simulink model "systune_darko"  (R2021b)
settings: Solver=VariableStepAuto  StartTime=0.0  StopTime=50  RelTol=1e-3
values from neighbouring files (symbols this model uses):
  C_control = [C(1:7,:);C(9:12,:)]    [main.m]
  drone = generateDarko()    [main.m]
  H_complet = solution(5:6,:)    [main.m]
  H_val = H_val.D    [main.m]
  initial_state = [p_initial; v_initial; q_initial; omega_initial]    [main.m]
  K_val = K_val.D    [main.m]
  Ki_complet = solution(1:4,:)    [main.m]
  u_eq_ = u_eq    [main.m]
  w = [0;0;0]    [main.m]
  x_eq_ = [[0; 0; 0]; [0; 0; 0]; [0; 0]; [0; 0; 0]]    [main.m]
libraries: simulink_extras x14, sharedtransform x2
settings Model: Creator=florian  LastModifiedBy=florian
settings SolverCC: AlgebraicLoopSolver=TrustRegion
settings DebuggingCC: SFMachineParentedDataDiag=warning

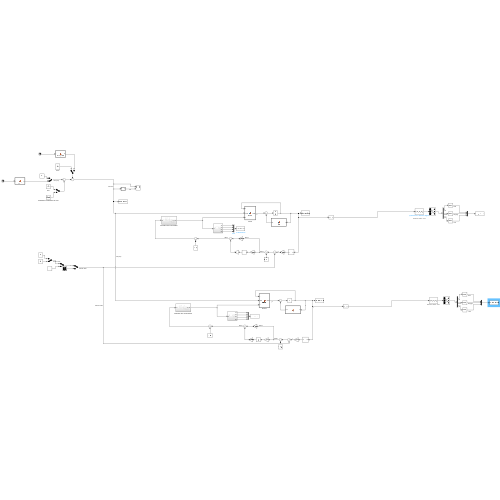
[thumbnail: Simulink's stored preview of the top-level diagram]
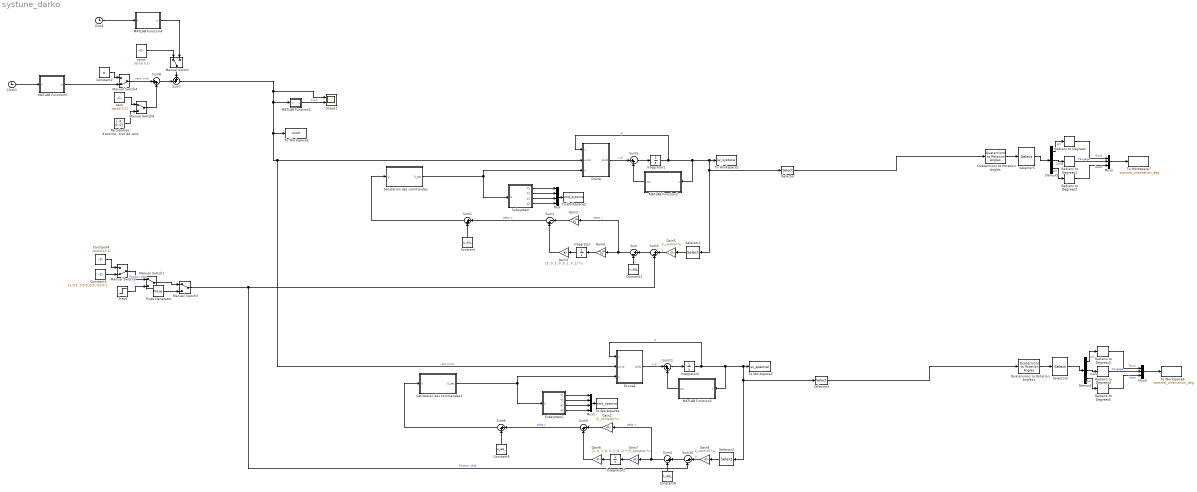
== system systune_darko ==
  Clock : Clock
  Clock1 : Clock
  Constant : Constant  Value=u_eq_
  Constant1 : Constant  Value=x_eq_
  Constant2 : Constant  Value=w
  Constant3 : Constant  Value=[1;0;1; 0;0;0; 0;0; 0;0;0;]
  Constant4 : Constant  Value=zeros(11,1)
  Constant5 : Constant  Value=u_eq_
  Constant6 : Constant  Value=x_eq_
  Demux1 : Demux  Outputs=3
  Demux5 : Demux  Outputs=3
  Drone : MATLAB Function  TreatAsAtomicUnit=on
  Drone1 : MATLAB Function  TreatAsAtomicUnit=on
  Gain1 : Gain  Gain=K_val  Multiplication=Matrix(K*u) (u vector)
  Gain2 : Gain  Gain=Ki_complet  Multiplication=Matrix(K*u) (u vector)
  Gain3 : Gain  Gain=[1, 0; 1, 0; 0, 1; 0, 1]  Multiplication=Matrix(K*u) (u vector)
  Gain4 : Gain  Gain=H_val  Multiplication=Matrix(K*u) (u vector)
  Gain5 : Gain  Gain=C_control  Multiplication=Matrix(K*u) (u vector)
  Gain6 : Gain  Gain=[1, 0; 1, 0; 0, 1; 0, 1]  Multiplication=Matrix(K*u) (u vector)
  Gain7 : Gain  Gain=H_complet  Multiplication=Matrix(K*u) (u vector)
  Gain8 : Gain  Gain=C_control  Multiplication=Matrix(K*u) (u vector)
  Integrator : Integrator  InitialCondition=zeros(1,2)
  Integrator1 : Integrator  InitialCondition=initial_state
  Integrator2 : Integrator  InitialCondition=zeros(1,2)
  Integrator3 : Integrator  InitialCondition=initial_state
  MATLAB Function1 : MATLAB Function  TreatAsAtomicUnit=on
  MATLAB Function2 : MATLAB Function  TreatAsAtomicUnit=on
  MATLAB Function3 : MATLAB Function  TreatAsAtomicUnit=on
  MATLAB Function4 : MATLAB Function  TreatAsAtomicUnit=on
  MATLAB Function5 : MATLAB Function  TreatAsAtomicUnit=on
  Manual Switch{,1,3,6} (4 alike) : ManualSwitch
  Manual Switch4 : ManualSwitch  CurrentSetting=0
  Manual Switch5 : ManualSwitch  CurrentSetting=0
  Mux : Mux
  Mux1 : Mux
  Mux2 : Mux  Inputs=3
  Mux3 : Mux  Inputs=3
  Pertubation d'estimation de vent : Constant  Value=[-3; 0; 0]
  Pulse Generator : DiscretePulseGenerator  PulseType=Time based  Amplitude=[0;0;-5; 0;0;0; 0;0; 0;0;0]  Period=5  PulseWidth=50
  Quaternions to Rotation Angles : sharedtransform/Quaternions to Rotation Angles  rotationOrder=ZXY  aMode=aMode
      settings: SourceProductBaseCode=AE,PW,DR,MT,UV,VE
  Quaternions to Rotation Angles1 : sharedtransform/Quaternions to Rotation Angles  rotationOrder=ZXY  aMode=aMode
      settings: SourceProductBaseCode=AE,PW,DR,MT,UV,VE
  Radians to Degrees{,1..5} (6 alike) : simulink_extras/Transformations/Radians to Degrees
  Satutation des commandes : Subsystem
  Satutation des commandes1 : Subsystem
  Scope1 : Scope  NumInputPorts=2
  Selector : Selector  InputPortWidth=13  IndexOptions=Index vector (dialog)  Indices=[7:10]  OutputSizes=1
  Selector1 : Selector  InputPortWidth=13  IndexOptions=Index vector (dialog)  Indices=[1:6 8:13]  OutputSizes=1
  Selector2 : Selector  InputPortWidth=13  IndexOptions=Index vector (dialog)  Indices=[1:6 8:13]  OutputSizes=1
  Selector3 : Selector  InputPortWidth=3  IndexOptions=Index vector (dialog)  Indices=[2 3 1]  OutputSizes=1
  Selector4 : Selector  InputPortWidth=13  IndexOptions=Index vector (dialog)  Indices=[7:10]  OutputSizes=1
  Selector5 : Selector  InputPortWidth=3  IndexOptions=Index vector (dialog)  Indices=[2 3 1]  OutputSizes=1
  Step1 : Step  Time=35  Before=zeros(11,1)  After=[-0.1;0;0; 0;0;0; 0;0; 0;0;0]  SampleTime=0
  Subsystem : Subsystem
  Subsystem1 : Subsystem
  Sum{,3..4,10} (4 alike) : Sum  Inputs=|+-
  Sum{1,5..6,8,11} (5 alike) : Sum  Inputs=|++
  Sum2 : Sum  Inputs=|-+
  Sum7 : Sum  Inputs=++|
  Sum9 : Sum  Inputs=|-+
  To Workspace1 : ToWorkspace  VariableName=sv_systune  SampleTime=-1
  To Workspace2 : ToWorkspace  VariableName=cmd_systune  SampleTime=-1
  To Workspace3 : ToWorkspace  VariableName=sv_spectral  SampleTime=-1
  To Workspace4 : ToWorkspace  VariableName=cmd_spectral  SampleTime=-1
  To Workspace5 : ToWorkspace  VariableName=wind  SampleTime=-1
  To Workspace6 : ToWorkspace  VariableName=spectral_orientation_deg  SampleTime=-1
  To Workspace7 : ToWorkspace  VariableName=systune_orientation_deg  SampleTime=-1
  zero : Constant  Value=zeros(3,1)
  zeros : Constant  Value=zeros(3,1)
  wires:
  Sum5/1 -> Integrator1/1
  MATLAB Function2/1(cor) -> Sum5/2
  Drone/1(dxdt) -> Sum5/1  "x_d"
  Constant1/1 -> Sum/2
  Sum1/1 -> Satutation des commandes/1(U)
  Integrator/1 -> Gain3/1
  Sum/1 -> Gain4/1, Gain1/1  "delta x"
  Gain4/1 -> Integrator/1
  Gain1/1 -> Sum2/1
  Selector1/1 -> Gain5/1
  Gain5/1 -> Sum3/1  "y"
  Sum3/1 -> Sum/1
  Gain3/1 -> Sum2/2
  MATLAB Function5/1(w) -> Manual Switch4/2
  Constant2/1 -> Manual Switch4/1
  MATLAB Function1/1(y) -> Scope1/2  "kmh"
  Step1/1 -> Manual Switch1/2
  Pulse Generator/1 -> Manual Switch3/2
  Manual Switch1/1 -> Manual Switch3/1
  Clock/1 -> MATLAB Function4/1(t)
  Constant3/1 -> Manual Switch5/2
  Manual Switch5/1 -> Manual Switch1/1  "Position cible"
  Constant4/1 -> Manual Switch5/1
  Integrator1/1 -> Drone/1(x), To Workspace1/1, Selector1/1, Selector/1, MATLAB Function2/1(x)  "p"
  Subsystem/1(T1) -> Mux/1
  Subsystem/3(d1) -> Mux/3
  Satutation des commandes/1(U_sat) -> Subsystem/1(U), Drone/3(u)
  Subsystem/2(T2) -> Mux/2
  Subsystem/4(d2) -> Mux/4
  Manual Switch/1 -> Sum7/1
  MATLAB Function4/1(w) -> Manual Switch/2
  zeros/1 -> Manual Switch/1
  Sum8/1 -> Sum7/2
  Manual Switch4/1 -> Sum8/1  "vent (m/s)"
  Pertubation d'estimation de vent/1 -> Manual Switch6/2
  Manual Switch6/1 -> Sum8/2
  zero/1 -> Manual Switch6/1
  Constant/1 -> Sum1/2
  Sum2/1 -> Sum1/1  "delta u"
  Mux/1 -> To Workspace2/1
  Subsystem1/2(T2) -> Mux1/2
  Sum4/1 -> Gain7/1, Gain2/1  "delta x"
  Drone1/1(dxdt) -> Sum11/1  "x_d"
  Sum11/1 -> Integrator3/1
  Manual Switch3/1 -> Sum3/2, Sum10/2  "Position cible"
  Selector2/1 -> Gain8/1
  Constant5/1 -> Sum6/2
  Integrator2/1 -> Gain6/1
  Satutation des commandes1/1(U_sat) -> Subsystem1/1(U), Drone1/3(u)
  Sum7/1 -> To Workspace5/1, Drone1/2(wind), Drone/2(wind), MATLAB Function1/1(u), Scope1/1  "vent (m/s)"
  Subsystem1/4(d2) -> Mux1/4
  Mux1/1 -> To Workspace4/1
  Subsystem1/3(d1) -> Mux1/3
  Subsystem1/1(T1) -> Mux1/1
  Gain6/1 -> Sum9/2
  Gain8/1 -> Sum10/1  "y"
  Constant6/1 -> Sum4/2
  MATLAB Function3/1(cor) -> Sum11/2
  Sum6/1 -> Satutation des commandes1/1(U)
  Gain2/1 -> Sum9/1
  Gain7/1 -> Integrator2/1
  Sum9/1 -> Sum6/1  "delta u"
  Sum10/1 -> Sum4/1
  Clock1/1 -> MATLAB Function5/1(t)
  Radians to Degrees/1 -> Mux2/1  "Rouli"
  Quaternions to Rotation Angles/1 -> Selector3/1
  Demux5/3 -> Radians to Degrees2/1  "psi"
  Demux5/2 -> Radians to Degrees1/1  "theta"
  Demux5/1 -> Radians to Degrees/1  "phi"
  Radians to Degrees1/1 -> Mux2/2  "Tangage"
  Selector/1 -> Quaternions to Rotation Angles/1
  Mux2/1 -> To Workspace7/1
  Radians to Degrees2/1 -> Mux2/3  "Lacet"
  Selector3/1 -> Demux5/1
  Radians to Degrees4/1 -> Mux3/2  "Tangage"
  Radians to Degrees3/1 -> Mux3/1  "Rouli"
  Selector4/1 -> Quaternions to Rotation Angles1/1
  Demux1/3 -> Radians to Degrees5/1  "psi"
  Selector5/1 -> Demux1/1
  Integrator3/1 -> Drone1/1(x), To Workspace3/1, Selector4/1, Selector2/1, MATLAB Function3/1(x)  "p"
  Radians to Degrees5/1 -> Mux3/3  "Lacet"
  Quaternions to Rotation Angles1/1 -> Selector5/1
  Mux3/1 -> To Workspace6/1
  Demux1/2 -> Radians to Degrees4/1  "theta"
  Demux1/1 -> Radians to Degrees3/1  "phi"

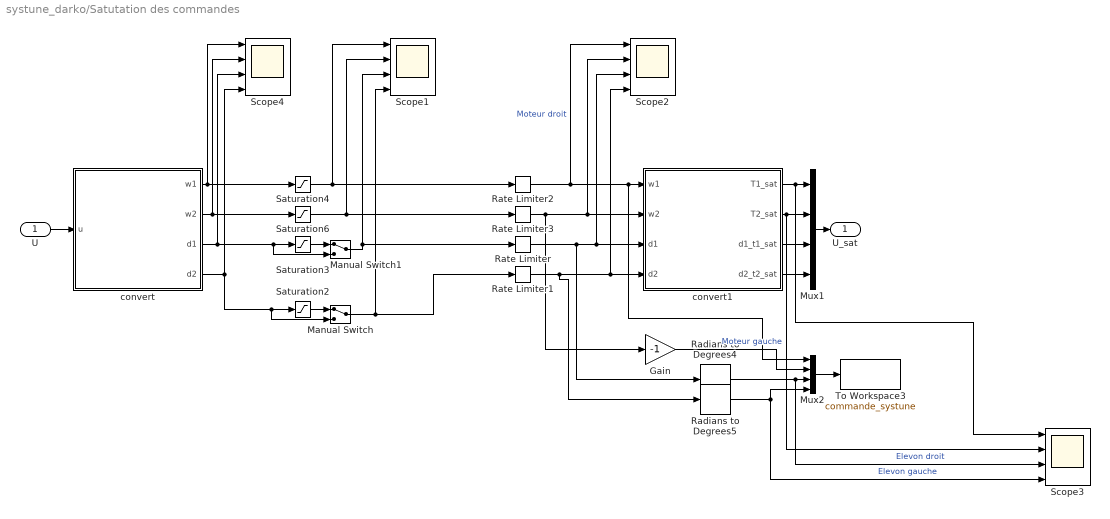
== system systune_darko/Satutation des commandes ==
  U : Inport
  Gain : Gain  Gain=-1
  Manual Switch : ManualSwitch
  Manual Switch1 : ManualSwitch
  Mux1 : Mux
  Mux2 : Mux
  Radians to Degrees4 : simulink_extras/Transformations/Radians to Degrees
  Radians to Degrees5 : simulink_extras/Transformations/Radians to Degrees
  Rate Limiter : RateLimiter  RisingSlewLimit=drone.ELEVON_RATE_CHANGE  FallingSlewLimit=-drone.ELEVON_RATE_CHANGE  SampleTimeMode=inherited
  Rate Limiter1 : RateLimiter  RisingSlewLimit=drone.ELEVON_RATE_CHANGE  FallingSlewLimit=-drone.ELEVON_RATE_CHANGE  SampleTimeMode=inherited
  Rate Limiter2 : RateLimiter  RisingSlewLimit=drone.MOTOR_RATE_CHANGE  FallingSlewLimit=-drone.MOTOR_RATE_CHANGE  SampleTimeMode=inherited
  Rate Limiter3 : RateLimiter  RisingSlewLimit=drone.MOTOR_RATE_CHANGE  FallingSlewLimit=-drone.MOTOR_RATE_CHANGE  SampleTimeMode=inherited
  Saturation2 : Saturate  UpperLimit=30*(pi/180)  LowerLimit=-30*(pi/180)
  Saturation3 : Saturate  UpperLimit=30*(pi/180)  LowerLimit=-30*(pi/180)
  Saturation4 : Saturate  UpperLimit=2000  LowerLimit=200
  Saturation6 : Saturate  UpperLimit=2000  LowerLimit=200
  Scope{1..4} (4 alike) : Scope  NumInputPorts=4
  To Workspace3 : ToWorkspace  VariableName=commande_systune  SampleTime=-1
  convert : MATLAB Function  TreatAsAtomicUnit=on
  convert1 : MATLAB Function  TreatAsAtomicUnit=on
  U_sat : Outport
  wires:
  convert/1(w1) -> Saturation4/1, Scope4/1
  convert/2(w2) -> Scope4/2, Saturation6/1
  convert/3(d1) -> Scope4/3, Manual Switch1/2, Saturation3/1
  convert/4(d2) -> Manual Switch/2, Saturation2/1, Scope4/4
  convert1/1(T1_sat) -> Scope3/1, Mux1/1
  convert1/4(d2_t2_sat) -> Mux1/4
  Mux1/1 -> U_sat/1
  convert1/2(T2_sat) -> Scope3/2, Mux1/2
  convert1/3(d1_t1_sat) -> Mux1/3
  Saturation6/1 -> Rate Limiter3/1, Scope1/2
  Saturation4/1 -> Rate Limiter2/1, Scope1/1
  U/1 -> convert/1(u)
  Radians to Degrees5/1 -> Mux2/4, Scope3/4  "Elevon gauche"
  Rate Limiter3/1 -> Gain/1, convert1/2(w2), Scope2/2
  Rate Limiter1/1 -> Radians to Degrees5/1, Scope2/4, convert1/4(d2)
  Rate Limiter/1 -> Radians to Degrees4/1, Scope2/3, convert1/3(d1)
  Gain/1 -> Mux2/2  "Moteur gauche"
  Mux2/1 -> To Workspace3/1
  Radians to Degrees4/1 -> Scope3/3, Mux2/3  "Elevon droit"
  Rate Limiter2/1 -> Scope2/1, Mux2/1, convert1/1(w1)  "Moteur droit"
  Saturation3/1 -> Manual Switch1/1
  Manual Switch1/1 -> Rate Limiter/1, Scope1/3
  Saturation2/1 -> Manual Switch/1
  Manual Switch/1 -> Scope1/4, Rate Limiter1/1

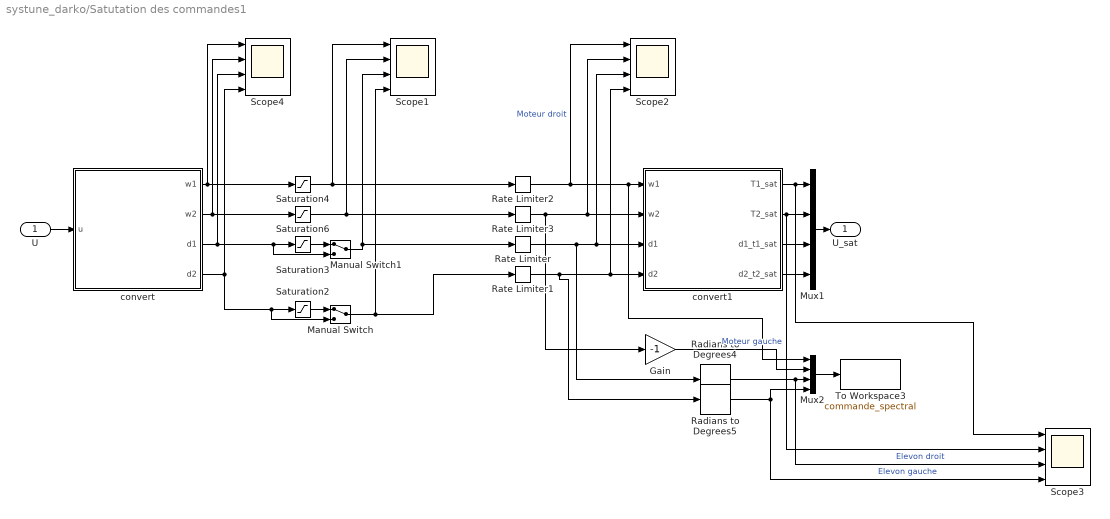
== system systune_darko/Satutation des commandes1 ==
  U : Inport
  Gain : Gain  Gain=-1
  Manual Switch : ManualSwitch
  Manual Switch1 : ManualSwitch
  Mux1 : Mux
  Mux2 : Mux
  Radians to Degrees4 : simulink_extras/Transformations/Radians to Degrees
  Radians to Degrees5 : simulink_extras/Transformations/Radians to Degrees
  Rate Limiter : RateLimiter  RisingSlewLimit=drone.ELEVON_RATE_CHANGE  FallingSlewLimit=-drone.ELEVON_RATE_CHANGE  SampleTimeMode=inherited
  Rate Limiter1 : RateLimiter  RisingSlewLimit=drone.ELEVON_RATE_CHANGE  FallingSlewLimit=-drone.ELEVON_RATE_CHANGE  SampleTimeMode=inherited
  Rate Limiter2 : RateLimiter  RisingSlewLimit=drone.MOTOR_RATE_CHANGE  FallingSlewLimit=-drone.MOTOR_RATE_CHANGE  SampleTimeMode=inherited
  Rate Limiter3 : RateLimiter  RisingSlewLimit=drone.MOTOR_RATE_CHANGE  FallingSlewLimit=-drone.MOTOR_RATE_CHANGE  SampleTimeMode=inherited
  Saturation2 : Saturate  UpperLimit=30*(pi/180)  LowerLimit=-30*(pi/180)
  Saturation3 : Saturate  UpperLimit=30*(pi/180)  LowerLimit=-30*(pi/180)
  Saturation4 : Saturate  UpperLimit=2000  LowerLimit=200
  Saturation6 : Saturate  UpperLimit=2000  LowerLimit=200
  Scope{1..4} (4 alike) : Scope  NumInputPorts=4
  To Workspace3 : ToWorkspace  VariableName=commande_spectral  SampleTime=-1
  convert : MATLAB Function  TreatAsAtomicUnit=on
  convert1 : MATLAB Function  TreatAsAtomicUnit=on
  U_sat : Outport
  wires:
  convert/1(w1) -> Saturation4/1, Scope4/1
  convert/2(w2) -> Scope4/2, Saturation6/1
  convert/3(d1) -> Scope4/3, Manual Switch1/2, Saturation3/1
  convert/4(d2) -> Manual Switch/2, Saturation2/1, Scope4/4
  convert1/1(T1_sat) -> Scope3/1, Mux1/1
  convert1/4(d2_t2_sat) -> Mux1/4
  Mux1/1 -> U_sat/1
  convert1/2(T2_sat) -> Scope3/2, Mux1/2
  convert1/3(d1_t1_sat) -> Mux1/3
  Saturation6/1 -> Rate Limiter3/1, Scope1/2
  Saturation4/1 -> Rate Limiter2/1, Scope1/1
  U/1 -> convert/1(u)
  Radians to Degrees5/1 -> Mux2/4, Scope3/4  "Elevon gauche"
  Rate Limiter3/1 -> Gain/1, convert1/2(w2), Scope2/2
  Rate Limiter1/1 -> Radians to Degrees5/1, Scope2/4, convert1/4(d2)
  Rate Limiter/1 -> Radians to Degrees4/1, Scope2/3, convert1/3(d1)
  Gain/1 -> Mux2/2  "Moteur gauche"
  Mux2/1 -> To Workspace3/1
  Radians to Degrees4/1 -> Scope3/3, Mux2/3  "Elevon droit"
  Rate Limiter2/1 -> Scope2/1, Mux2/1, convert1/1(w1)  "Moteur droit"
  Saturation3/1 -> Manual Switch1/1
  Manual Switch1/1 -> Rate Limiter/1, Scope1/3
  Saturation2/1 -> Manual Switch/1
  Manual Switch/1 -> Scope1/4, Rate Limiter1/1

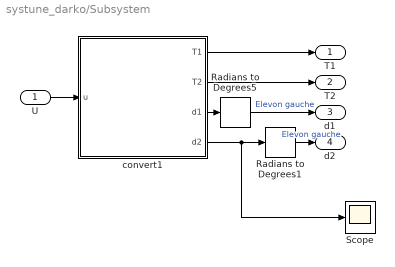
== system systune_darko/Subsystem ==
  U : Inport
  Radians to Degrees1 : simulink_extras/Transformations/Radians to Degrees
  Radians to Degrees5 : simulink_extras/Transformations/Radians to Degrees
  Scope : Scope
  convert1 : MATLAB Function  TreatAsAtomicUnit=on
  T1 : Outport
  T2 : Outport  Port=2
  d1 : Outport  Port=3
  d2 : Outport  Port=4
  wires:
  U/1 -> convert1/1(u)
  convert1/1(T1) -> T1/1
  convert1/2(T2) -> T2/1
  Radians to Degrees5/1 -> d1/1  "Elevon gauche"
  convert1/3(d1) -> Radians to Degrees5/1
  Radians to Degrees1/1 -> d2/1  "Elevon gauche"
  convert1/4(d2) -> Scope/1, Radians to Degrees1/1

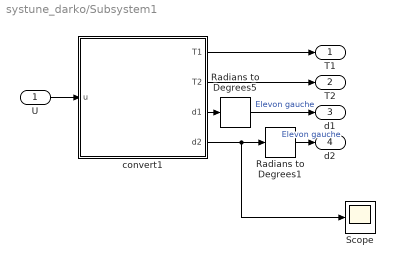
== system systune_darko/Subsystem1 ==
  U : Inport
  Radians to Degrees1 : simulink_extras/Transformations/Radians to Degrees
  Radians to Degrees5 : simulink_extras/Transformations/Radians to Degrees
  Scope : Scope
  convert1 : MATLAB Function  TreatAsAtomicUnit=on
  T1 : Outport
  T2 : Outport  Port=2
  d1 : Outport  Port=3
  d2 : Outport  Port=4
  wires:
  U/1 -> convert1/1(u)
  convert1/1(T1) -> T1/1
  convert1/2(T2) -> T2/1
  Radians to Degrees5/1 -> d1/1  "Elevon gauche"
  convert1/3(d1) -> Radians to Degrees5/1
  Radians to Degrees1/1 -> d2/1  "Elevon gauche"
  convert1/4(d2) -> Scope/1, Radians to Degrees1/1

== matlab function systune_darko/Satutation des commandes/convert ==
  data: u input; w1 output; drone parameter; w2 output; d1 output; d2 output
function [w1, w2, d1, d2] = convert(u, drone)
%#codegen
kf = drone.PROP_KP;

T1 = max(u(1),0);
T2 = max(u(2),0);
d1 = u(3);
d2 = u(4);

w1 = sqrt(T1/kf);
w2 = sqrt(T2/kf);

== matlab function systune_darko/MATLAB Function5 ==
  data: t input; w output
function w = step_wind(t)
%#codegen

if t<=15 
    wx = 0;
elseif t>15 && t<=30
    wx = 1;
elseif t>30 && t<=45
    wx = 2;
elseif t>45 && t<=60
    wx = 3;
else
    wx = 4;
end
w = [-wx;0;0];

== matlab function systune_darko/Satutation des commandes/convert1 ==
  data: w1 input; w2 input; d1 input; d2 input; T1_sat output; T2_sat output; drone parameter; d1_t1_sat output; d2_t2_sat output
function [T1_sat, T2_sat, d1_t1_sat, d2_t2_sat] = convert2(w1, w2, d1, d2, drone)
%#codegen
kf = drone.PROP_KP;

T1_sat = kf*w1^2;
d1_t1_sat = d1*T1_sat;
T2_sat = kf*w2^2;
d2_t2_sat = d2*T2_sat;

== matlab function systune_darko/MATLAB Function2 ==
  data: x input; cor output
function cor  = fcn(x)
%#codegen
q  = x(7:10);
n = norm(q);
mismatch = 1-n;
cor = [0;0;0; 0;0;0; mismatch*q; 0;0;0];

== matlab function systune_darko/Drone1 ==
  data: x input; wind input; u input; dxdt output; drone parameter
function dxdt  = drone(x,wind, u, drone)

%% physical constants
% gravity
g = drone.G;
% vehicle mass
m = drone.MASS;
% vehicle inertia matrix
J = drone.INERTIA; % [3x3 real symmetric] in body axis

%% state demultiplexing
% p = x(1:3);
v = x(4:6);
q  = x(7:10);
wb = x(11:13);

Rq = q2dcm(q);

[Fp, Mp] = external_force_moment(x, u, wind, drone);

% position
dpdt = v;

% kinematics
dvdt =  [0;0;g] + (1/m)*Rq*drone.Fb*u + (1/m)*Rq*Fp; 

%% quaternion derivative
eta = q(1);
eps = q(2:4);

dqdt = (1/2)*[-eps'; eta*eye(3) + skew_sym(eps)]*wb;

%% angular velocity derivative
% kinematics
dwdt = -J\cross(wb, J*wb) + J\(drone.Mb*u) + J\Mp;


%% derivative multiplexing
dxdt = [dpdt; dvdt; dqdt; dwdt] ;

== matlab function systune_darko/Drone ==
  data: x input; wind input; u input; dxdt output; drone parameter
function dxdt  = drone(x,wind, u, drone)

%% physical constants
% gravity
g = drone.G;
% vehicle mass
m = drone.MASS;
% vehicle inertia matrix
J = drone.INERTIA; % [3x3 real symmetric] in body axis

%% state demultiplexing
% p = x(1:3);
v = x(4:6);
q  = x(7:10);
wb = x(11:13);

Rq = q2dcm(q);

[Fp, Mp] = external_force_moment(x, u, wind, drone);

% position
dpdt = v;

% kinematics
dvdt =  [0;0;g] + (1/m)*Rq*drone.Fb*u + (1/m)*Rq*Fp; 

%% quaternion derivative
eta = q(1);
eps = q(2:4);

dqdt = (1/2)*[-eps'; eta*eye(3) + skew_sym(eps)]*wb;

%% angular velocity derivative
% kinematics
dwdt = -J\cross(wb, J*wb) + J\(drone.Mb*u) + J\Mp;


%% derivative multiplexing
dxdt = [dpdt; dvdt; dqdt; dwdt] ;

== matlab function systune_darko/Subsystem/convert1 ==
  data: u input; T1 output; drone parameter; T2 output; d1 output; d2 output
function [T1, T2, d1, d2] = convert(u, drone)
%#codegen
kf = drone.PROP_KP;

T1 = max(u(1),0);
T2 = max(u(2),0);
d1_T1 = u(3);
d2_T2 = u(4);

w1 = sqrt(T1/kf);
w2 = sqrt(T2/kf);
d1 = d1_T1/T1;
d2 = d2_T2/T2;

== matlab function systune_darko/MATLAB Function1 ==
  data: u input; y output
function y = nor(u)
%#codegen

y = norm(u)*3.6;

== matlab function systune_darko/MATLAB Function4 ==
  data: t input; w output
function w = mex_wind(t)
%#codegen
t0 = 20; %s
wx_mean = 0;
fg = 0.8;
Ag = -1; %m/s
if (t-t0)<0 ||  (t-t0)> 1/fg
    wx = wx_mean;
else
    wx = wx_mean + (Ag/2)*(1-cos(2*pi*fg*(t-t0)))*sin(3*pi*fg*(t-t0));
end
w = [-wx;0;0];

== matlab function systune_darko/MATLAB Function3 ==
  data: x input; cor output
function cor  = fcn(x)
%#codegen
q  = x(7:10);
n = norm(q);
mismatch = 1-n;
cor = [0;0;0; 0;0;0; mismatch*q; 0;0;0];

== matlab function systune_darko/Satutation des commandes1/convert ==
  data: u input; w1 output; drone parameter; w2 output; d1 output; d2 output
function [w1, w2, d1, d2] = convert(u, drone)
%#codegen
kf = drone.PROP_KP;

T1 = max(u(1),0);
T2 = max(u(2),0);
d1 = u(3);
d2 = u(4);

w1 = sqrt(T1/kf);
w2 = sqrt(T2/kf);

== matlab function systune_darko/Satutation des commandes1/convert1 ==
  data: w1 input; w2 input; d1 input; d2 input; T1_sat output; T2_sat output; drone parameter; d1_t1_sat output; d2_t2_sat output
function [T1_sat, T2_sat, d1_t1_sat, d2_t2_sat] = convert2(w1, w2, d1, d2, drone)
%#codegen
kf = drone.PROP_KP;

T1_sat = kf*w1^2;
d1_t1_sat = d1*T1_sat;
T2_sat = kf*w2^2;
d2_t2_sat = d2*T2_sat;

== matlab function systune_darko/Subsystem1/convert1 ==
  data: u input; T1 output; drone parameter; T2 output; d1 output; d2 output
function [T1, T2, d1, d2] = convert(u, drone)
%#codegen
kf = drone.PROP_KP;

T1 = max(u(1),0);
T2 = max(u(2),0);
d1_T1 = u(3);
d2_T2 = u(4);

w1 = sqrt(T1/kf);
w2 = sqrt(T2/kf);
d1 = d1_T1/T1;
d2 = d2_T2/T2;
